simulink model "spacecraft3"  (R2021a)
settings: Solver=ode45  StartTime=0.0  StopTime=27000  RelTol=1e-12  AbsTol=1e-12
settings Model: Creator=fg7823  LastModifiedBy=fg7823

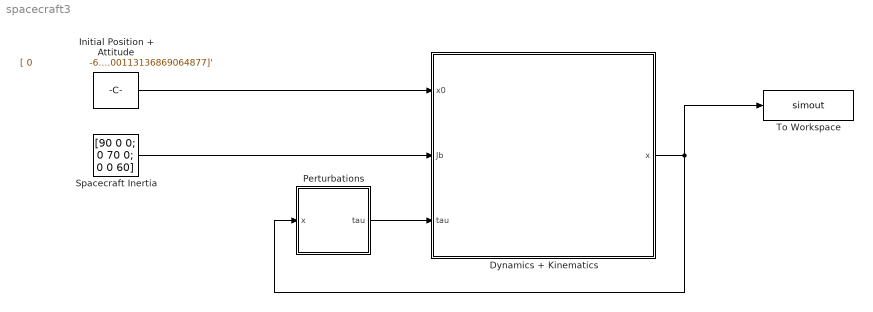
== system spacecraft3 ==
  Dynamics + Kinematics : Subsystem
  Initial Position + Attitude : Constant  Value=|
      | [ 0
      |                   -6778137
      |                          0
      |           7668.57198272798
      |      0
      |                          0
      |                          0
      |                          0
      |      0
      |                          1
      |       1.74532925199433e-06
      |       1.74532925199433e-06
      |        0.00113136869064877]'
  Perturbations : Subsystem
  Spacecraft Inertia : Constant  Value=[90 0 0; 0 70 0; 0 0 60]
  To Workspace : ToWorkspace  VariableName=simout  SampleTime=-1
  wires:
  Spacecraft Inertia/1 -> Dynamics + Kinematics/2(Jb)
  Initial Position + Attitude/1 -> Dynamics + Kinematics/1(x0)
  Dynamics + Kinematics/1(x) -> To Workspace/1, Perturbations/1(x)
  Perturbations/1(tau) -> Dynamics + Kinematics/3(tau)

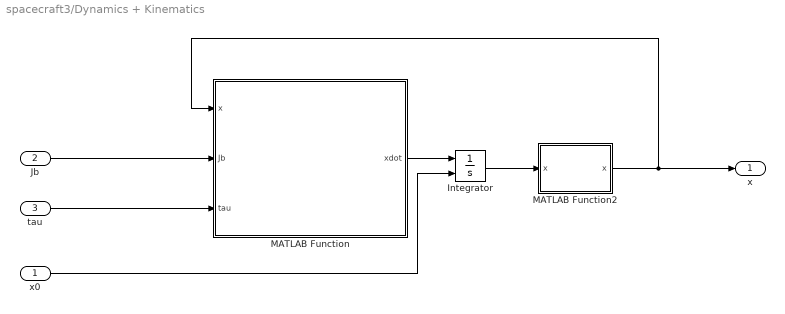
== system spacecraft3/Dynamics + Kinematics ==
  x0 : Inport
  Jb : Inport  Port=2
  tau : Inport  Port=3
  Integrator : Integrator  InitialConditionSource=external
  MATLAB Function : MATLAB Function  TreatAsAtomicUnit=on
  MATLAB Function2 : MATLAB Function  TreatAsAtomicUnit=on
  x : Outport
  wires:
  Jb/1 -> MATLAB Function/2(Jb)
  x0/1 -> Integrator/2
  MATLAB Function/1(xdot) -> Integrator/1
  tau/1 -> MATLAB Function/3(tau)
  Integrator/1 -> MATLAB Function2/1("x ")
  MATLAB Function2/1(x) -> x/1, MATLAB Function/1(x)

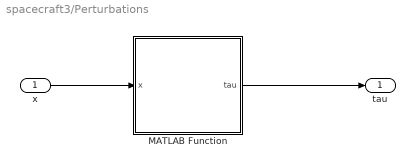
== system spacecraft3/Perturbations ==
  x : Inport
  MATLAB Function : MATLAB Function  TreatAsAtomicUnit=on
  tau : Outport
  wires:
  x/1 -> MATLAB Function/1(x)
  MATLAB Function/1(tau) -> tau/1

== matlab function spacecraft3/Dynamics + Kinematics/MATLAB Function ==
  data: x input; xdot output; Jb input; tau input
function xdot = propagation(x,Jb,tau)
    G           = 6.6743e-11;                    % m3/kgs2
    m_e         = 5.97219e+24;   
    % Unpacking states
    ri          = x(1:3);
    vi          = x(4:6);
    qb_i        = x(7:10);
    wb_bi       = x(11:13);
    xdot        = zeros(13,1);
    % Propagation of position & velocity 
    xdot(1:3)   = vi;
    xdot(4:6)   = -G*m_e*ri/(norm(ri)^3);
    % Propagation of kinematics
    xdot(7:10)  = otimes([wb_bi; 0],qb_i)/2;
    % Propagation of dynamics
    xdot(11:13) = inv(Jb)*(-cross(wb_bi,Jb*wb_bi) + tau);
end

== matlab function spacecraft3/Dynamics + Kinematics/MATLAB Function2 ==
  data: x input; x output
function x = normalize(x)
     x(7:10) = x(7:10)/norm(x(7:10));
end

== matlab function spacecraft3/Perturbations/MATLAB Function ==
  data: x input; tau output
function tau = aerodynamic(x)

    % Intrinsic values
    w_e   = 2*pi/(24*60*60);
    w_e   = [0; 0; w_e];
    
    rho0  = 3.725e-12;   
    r_e   = 6378e3; 
    H     = 58.515e3;
    
    % Unpacking state
    ri    = x(1:3);
    vi    = x(4:6);
    qb_i  = x(7:10);
    
    % Solar panel parameters
    nb  = [1 0 0]';
    A   = 1;
    cpb = [0 0 1.5]';
    Cd  = 2;
    
    vreli = vi - cross(w_e,ri);
    vrelb = Tq(qb_i)*vreli;
    
    rho  = rho0*exp(-((norm(ri)-r_e)-400e3)/H);
    fb   = -rho*A*Cd*((vrelb'*nb)^2)*(vrelb/norm(vrelb))/2;
    tau  = cross(cpb,fb);
end
